simulink model "BarrelControl"  (R2020b)
settings: Solver=VariableStepAuto  StartTime=0.0  StopTime=100  RelTol=1e-3
model workspace (MAT data in the model file):
  C = [0.75  -0.125  -0.5625  0.96875  -0.890625  0.3671875  0.33984375; 1  0  0  0  0  0  0; 0  1  0  0  0  0  0; 0  0  1  0  0  0  0; 0  0  0  1  0  0  0; 0  0  0  0  1  0  0; 0  0  0  0  0  1  0; 0  0  0  0  0  0  1]
  F2Q_xi0 = [1; -1; 1; -1; 1; -1; 1; -1]
  F2Q_xiL = [1; -1; 1; -1; 1; -1; 1; -1]
  Fg = [-29.43; 0; 9.81; 0; 1.962; 0; 0.840857142857; 0]
  Gama = [0  0  0  0  0  0  0; 0  30.2447027552  0  0  0  0  0; 0  0  91.5476694177  0  0  0  0; 0  0  0  175.64612088  0  0  0; 0  0  0  0  277.957713504  0  0; 0  0  0  0  0  1100.88467044  0; 0  0  0  0  0  0  2038.12753726]
  L = 3
  Lambda = [0  0  0  0  0  0  0; 0  91474.204475  0  0  0  0  0; 0  0  838097.577581  0  0  0  0; 0  0  0  3085155.97801  0  0  0; 0  0  0  0  7726049.04966  0  0; 0  0  0  0  0  121194705.761  0; 0  0  0  0  0  0  415396385.815]
  M2Q_xi0 = [0; 0.666666666667; -2.66666666667; 6; -10.6666666667; 16.6666666667; -24; 32.6666666667]
  PHI = [0.136866267704  0.0929914914005  -0.0980787352338  0.0555043868032  -0.144825832461  0.000118902872906  0.118435530445; 0  0.176249339781  -0.0244216885495  -0.133658178847  -0.00189383847447  0.12060390182  0.00720960774598; 0  0.00349791805609  -0.176715791557  -0.00267551593374  -0.105734711917  0.0527964768773  0.110849023327; 0  -0.0152299946368  -0.00490735942162  -0.149265467727  -0.0644504660459  0.117016733417  0.0261303448738; 0  -0.000276595902476  0.0380667589498  0.00904195510557  -0.127293898603  0.0724116243586  0.141528738637; 0  0.00125236425091  0.00154131438463  0.0381220764691  0.018603663864  0.181452010974  0.0171982021012; 0  -6.40906127314e-05  -0.00446596070835  -0.00233149354725  0.0468542529712  0.00391723696732  0.191561402886]
  dpsi_0 = [0; 0.666666666667; -2.66666666667; 6; -10.6666666667; 16.6666666667; -24; 32.6666666667]
  dpsi_L = [0; 0.666666666667; 2.66666666667; 6; 10.6666666667; 16.6666666667; 24; 32.6666666667]
  dpsi_Ldiv8 = [0; 0.666666666667; -2; 2.5; -1; -2.29166666667; 5.625; -6.63541666667]
  psi_0 = [1; -1; 1; -1; 1; -1; 1; -1]
  psi_L = [1; 1; 1; 1; 1; 1; 1; 1]
  ts_controller = 0.001
undefined symbols (not defined in the file): Theta
libraries: cstblocks x4, pid_lib x3, slctrlblks x1, simulink x1
settings Model: EnablePacing=on  OrderedModelArguments=off  Creator=alons  LastModifiedBy=alons

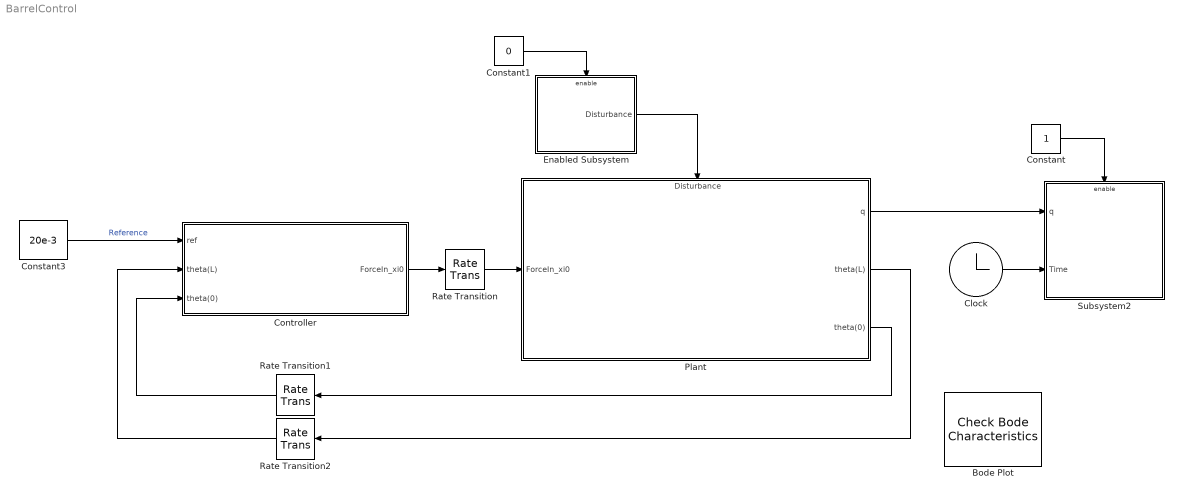
== system BarrelControl ==
  Bode Plot : slctrlblks/Model Verification/Check Bode  Characteristics  InstantiateOnLoad=on  SaveOperatingPoints=off  LinearizationIOs={'/Rate Transition', 1, 'in', 'on', '';'/Plant', 3, 'out', 'on', ''}  LinearizeAt=SnapshotTimes  SnapshotTimes=[0]  TriggerType=rising  SampleTime=auto  RateConversionMethod=zoh  PreWarpFreq=10  UseExactDelayModel=off  UseFullBlockNameLabels=off  UseBusSignalLabels=off  enabled=on  stopWhenAssertionFail=off  export=off  ViewDlgPos=[100 110.6 941 479.4]  OpenViewOnLoad=on  LaunchViewOnOpen=off  FrequencyUnits=rad/s  MagnitudeUnits=dB  PhaseUnits=deg  TimeUnits=seconds  EnableUpperBound=off  UpperBoundFrequencies=[]  UpperBoundMagnitudes=[]  EnableLowerBound=off  LowerBoundFrequencies=[]  LowerBoundMagnitudes=[]
  Clock : Clock
  Constant : Constant  SampleTime=0
      settings: OpenFcn=|
      | if get_param(gcbh,'value')-48
      |    set_param(gcbh,'value','0','backgroundcolor','red');
      | else
      |    set_param(gcbh,'value','1','backgroundcolor','green');
      | end
  Constant1 : Constant  Value=0  SampleTime=0
      settings: OpenFcn=|
      | if get_param(gcbh,'value')-48
      |    set_param(gcbh,'value','0','backgroundcolor','red');
      | else
      |    set_param(gcbh,'value','1','backgroundcolor','green');
      | end
  Constant3 : Constant  Value=20e-3
  Controller : Subsystem  Variant=on  VariantControlMode=label  VariantControl=Choice  LabelModeActiveChoice=Theta(0)
  Enabled Subsystem : Subsystem  TreatAsAtomicUnit=on
  Plant : Subsystem  TreatAsAtomicUnit=on
      settings: PortSchema="{\"entries\":[{\"content\":{\"sides\":[{\"content\":{\"connectorIds\":[\"In1\"]},\"type\":\"ConnectorPlacement.EquallySpacedRectSide\",\"uuid\":\"36edcb47-3a13-438a-ad6c-79b402161546\"},{\"content\":{\"connectorIds\":[\"Out1\",\"Out2\",\"Out3\"],\"side\":\"RIGHT\"},\"type\":\"ConnectorPlacement.EquallySpacedRectSide\",\"uuid\":\"f206446b-0714-4d39-be89-dc03dcd153f7\"},{\"content\":{\"connectorIds\":[\"In2\"],\"side\":\"TOP\"},\"type\":\"ConnectorPlacement.EquallySpacedRectSide\",\"uuid\":\"bd075090-b99d-4803-89e5-3bedf44d599a\"},{\"content\":{\"connectorIds\":[],\"side\":\"HIDDEN\"},\"type\":\"ConnectorPlacement.EquallySpacedRectSide\",\"uuid\":\"510f68a2-1cb4-4401-810b-32bb3d0b381d\"}]},\"type\":\"ConnectorPlacement.EquallySpacedConnector\",\"uuid\":\"6436aeff-31cc-4ec9-a090-95bfbf49f0cf\"}],\"packageUris\":[\"http://schema.mathworks.com/mf0/Connector/R2020b\"],\"version\":\"1.0\"}"
  Rate Transition : RateTransition
  Rate Transition1 : RateTransition  OutPortSampleTime=ts_controller
  Rate Transition2 : RateTransition  OutPortSampleTime=ts_controller
  Subsystem2 : Subsystem
      settings: OpenFcn=|
      | UserData = get_param([gcb,'/AnimationSfcn'],'UserData');
      | Fig = UserData.Figure;
      | if ishghandle(Fig,'figure');
      |    %bring to the front:
      |    figure(Fig);
      | end
      mask Display:
      | t=linspace(0,2*pi,20);
      | plot(cos(t),sin(t));
      | 
      | x=[-0.4,-0.4,0.6,-0.4];
      | y=[-0.5,0.5,0,-0.5];
      | plot(x,y)
      | 
      | color('black');
      | disp('Plot Beam');
  wires:
  Clock/1 -> Subsystem2/2(Time)
  Constant/1 -> Subsystem2/Enable
  Plant/1(q) -> Subsystem2/1(q)
  Plant/2(theta(L)) -> Rate Transition2/1
  Plant/3(theta(0)) -> Rate Transition1/1
  Rate Transition/1 -> Plant/1(ForceIn_xi0)
  Constant3/1 -> Controller/1(ref)  "Reference"
  Rate Transition2/1 -> Controller/2(theta(L))
  Rate Transition1/1 -> Controller/3(theta(0))
  Constant1/1 -> Enabled Subsystem/Enable
  Enabled Subsystem/1(Disturbance) -> Plant/2(Disturbance)
  Controller/1(ForceIn_xi0) -> Rate Transition/1

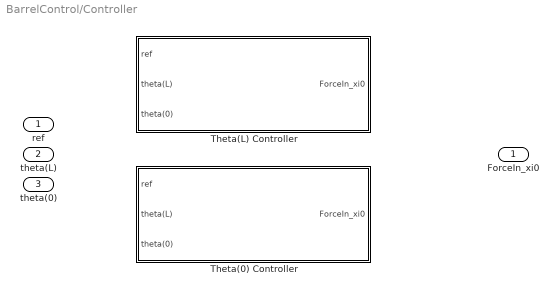
== system BarrelControl/Controller ==
  ref : Inport
  theta(L) : Inport  Port=2
  theta(0) : Inport  Port=3
  Theta(0) Controller : Subsystem  TreatAsAtomicUnit=on  VariantControl=Theta(0)
  Theta(L) Controller : Subsystem  TreatAsAtomicUnit=on  VariantControl=Theta(L)
  ForceIn_xi0 : Outport

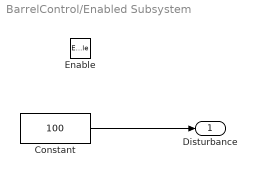
== system BarrelControl/Enabled Subsystem ==
  Enable : EnablePort  StatesWhenEnabling=reset
  Constant : Constant  Value=100
  Disturbance : Outport  OutputWhenDisabled=reset  InitialOutput=0
  wires:
  Constant/1 -> Disturbance/1

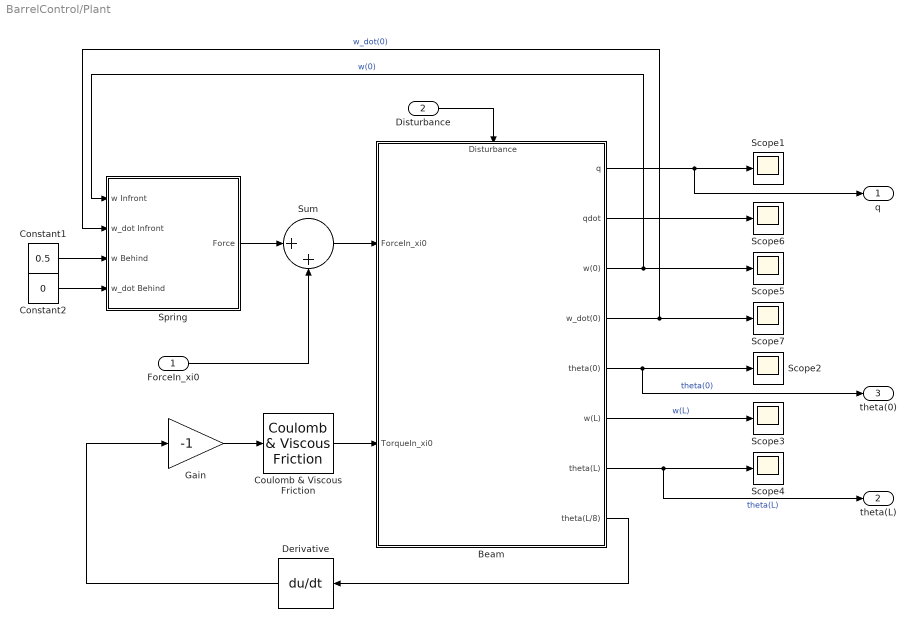
== system BarrelControl/Plant ==
  ForceIn_xi0 : Inport
  Disturbance : Inport  Port=2
  Beam : Subsystem
      settings: PortSchema="{\"entries\":[{\"content\":{\"sides\":[{\"content\":{\"connectorIds\":[\"In1\",\"In2\"]},\"type\":\"ConnectorPlacement.EquallySpacedRectSide\",\"uuid\":\"abe6467a-2196-4326-b3df-78fc9ab57750\"},{\"content\":{\"connectorIds\":[\"Out1\",\"Out2\",\"Out3\",\"Out4\",\"Out5\",\"Out6\",\"Out7\",\"Out8\"],\"side\":\"RIGHT\"},\"type\":\"ConnectorPlacement.EquallySpacedRectSide\",\"uuid\":\"8f33c77a-829a-46db-9e71-a7c761c5b10e\"},{\"content\":{\"connectorIds\":[\"In3\"],\"side\":\"TOP\"},\"type\":\"ConnectorPlacement.EquallySpacedRectSide\",\"uuid\":\"f7becae8-30ec-4352-b968-96f4fe9b45e3\"},{\"content\":{\"connectorIds\":[],\"side\":\"HIDDEN\"},\"type\":\"ConnectorPlacement.EquallySpacedRectSide\",\"uuid\":\"eaf9c01e-636e-4137-bd85-9b7716ad4e28\"}]},\"type\":\"ConnectorPlacement.EquallySpacedConnector\",\"uuid\":\"f90a8ce3-a2cb-42eb-a052-d6f5b77e739e\"}],\"packageUris\":[\"http://schema.mathworks.com/mf0/Connector/R2020b\"],\"version\":\"1.0\"}"
  Constant1 : Constant  Value=0.5
  Constant2 : Constant  Value=0
  Coulomb & Viscous Friction : simulink/Discontinuities/Coulomb & Viscous Friction  offset=15  gain=200
  Derivative : Derivative
  Gain : Gain  Gain=-1
  Scope{1..7} (7 alike) : Scope
  Spring : Subsystem
      mask Display: disp('Spring')
  Sum : Sum  Inputs=|++
  q : Outport
  theta(L) : Outport  Port=2
  theta(0) : Outport  Port=3
  wires:
  Beam/1(q) -> q/1, Scope1/1
  Constant1/1 -> Spring/3(w Behind)
  Beam/2(qdot) -> Scope6/1
  Sum/1 -> Beam/1(ForceIn_xi0)
  Beam/6(w(L)) -> Scope3/1  "w(L)"
  Constant2/1 -> Spring/4(w_dot Behind)
  Spring/1(Force) -> Sum/1
  Beam/3(w(0)) -> Spring/1(w Infront), Scope5/1  "w(0)"
  Beam/7(theta(L)) -> theta(L)/1, Scope4/1  "theta(L)"
  Beam/5(theta(0)) -> theta(0)/1, Scope2/1  "theta(0)"
  Beam/4(w_dot(0)) -> Spring/2(w_dot Infront), Scope7/1  "w_dot(0)"
  Coulomb & Viscous Friction/1 -> Beam/2(TorqueIn_xi0)
  ForceIn_xi0/1 -> Sum/2
  Disturbance/1 -> Beam/3(Disturbance)
  Gain/1 -> Coulomb & Viscous Friction/1
  Beam/8(theta(L/8)) -> Derivative/1
  Derivative/1 -> Gain/1

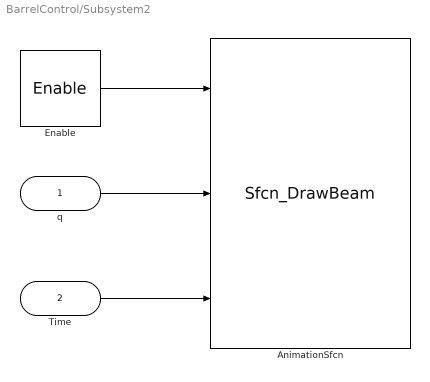
== system BarrelControl/Subsystem2 ==
  q : Inport
  Time : Inport  Port=2
  Enable : EnablePort  StatesWhenEnabling=reset  ShowOutputPort=on
  AnimationSfcn : M-S-Function  FunctionName=Sfcn_DrawBeam  Parameters=L
  wires:
  q/1 -> AnimationSfcn/2
  Enable/1 -> AnimationSfcn/1
  Time/1 -> AnimationSfcn/3

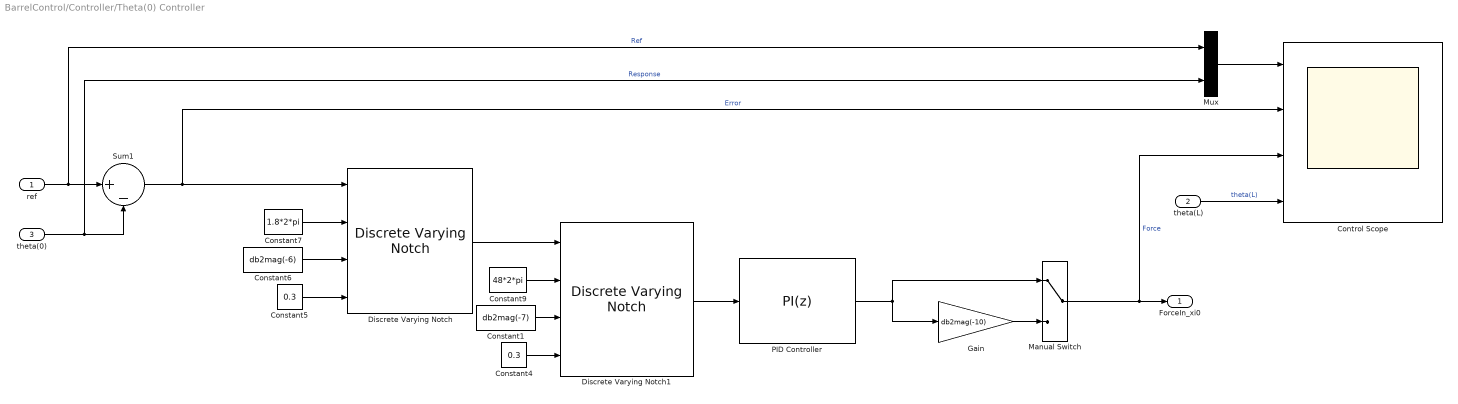
== system BarrelControl/Controller/Theta(0) Controller ==
  ref : Inport
  theta(L) : Inport  Port=2
  theta(0) : Inport  Port=3
  Constant1 : Constant  Value=db2mag(-7)
  Constant4 : Constant  Value=0.3
  Constant5 : Constant  Value=0.3
  Constant6 : Constant  Value=db2mag(-6)
  Constant7 : Constant  Value=1.8*2*pi
  Constant9 : Constant  Value=48*2*pi
  Control Scope : Scope  NumInputPorts=4
  Discrete Varying Notch : cstblocks/Linear Parameter Varying/Discrete Varying Notch  w0=1.5*2*pi  Ts=ts_controller
      settings: SourceProductBaseCode=CT
  Discrete Varying Notch1 : cstblocks/Linear Parameter Varying/Discrete Varying Notch  w0=48*2*pi  Ts=ts_controller
      settings: SourceProductBaseCode=CT
  Gain : Gain  Gain=db2mag(-10)
  Manual Switch : ManualSwitch
  Mux : Mux  Inputs=2
  PID Controller : pid_lib/PID Controller  Controller=PI  Form=Parallel  TimeDomain=Discrete-time  UseExternalTs=off  SampleTime=-1  IntegratorMethod=Forward Euler  FilterMethod=Forward Euler  ControllerParametersSource=internal  P=-9986.27949385  I=-157091.308648994  D=0  UseFilter=on  N=100  TunerSelectOption=Transfer Function Based (PID Tuner App)  InitialConditionSource=internal  InitialConditionForIntegrator=0  InitialConditionForFilter=0  DifferentiatorICPrevScaledInput=0  ExternalReset=none  TrackingMode=off  Kt=1  LimitOutput=off  SatLimitsSource=internal  UpperSaturationLimit=inf  LowerSaturationLimit=-inf  LinearizeAsGain=on  AntiWindupMode=none  Kb=1  POutMin=[]  POutMax=[]  IOutMin=[]  IOutMax=[]  DOutMin=[]  DOutMax=[]  NOutMin=[]  NOutMax=[]  SumOutMin=[]  SumOutMax=[]  SaturationOutMin=[]  SaturationOutMax=[]  PParamMin=[]  PParamMax=[]  IParamMin=[]  IParamMax=[]  DParamMin=[]  DParamMax=[]  NParamMin=[]  NParamMax=[]  KbParamMin=[]  KbParamMax=[]  KtParamMin=[]  KtParamMax=[]  KbOutMin=[]  KbOutMax=[]  KtOutMin=[]  KtOutMax=[]  IntegratorOutMin=[]  IntegratorOutMax=[]  FilterOutMin=[]  FilterOutMax=[]  SumI1OutMin=[]  SumI1OutMax=[]  SumI2OutMin=[]  SumI2OutMax=[]  SumI3OutMin=[]  SumI3OutMax=[]  SumI4OutMin=[]  SumI4OutMax=[]  SumDOutMin=[]  SumDOutMax=[]  DifferentiatorOutMin=[]  DifferentiatorOutMax=[]  FilterDiffOutCoefMin=[]  FilterDiffOutCoefMax=[]  ReciprocalOutMin=[]  ReciprocalOutMax=[]  SumDenOutMin=[]  SumDenOutMax=[]  SumNumOutMin=[]  SumNumOutMax=[]  DivideOutMin=[]  DivideOutMax=[]  UdiffTsProdOutMin=[]  UdiffTsProdOutMax=[]  NTsProdOutMin=[]  NTsProdOutMax=[]  UintegralTsProdOutMin=[]  UintegralTsProdOutMax=[]  UngainTsProdOutMin=[]  UngainTsProdOutMax=[]  IntegratorContinuousStateAttributes=''  IntegratorStateMustResolveToSignalObject=off  IntegratorRTWStateStorageClass=Auto  FilterContinuousStateAttributes=''  FilterStateMustResolveToSignalObject=off  FilterRTWStateStorageClass=Auto  ParallelPVariant=InternalParameters  IdealPVariant=Disabled  IVariant=InternalParameters  DVariant=Disabled  IntegratorVariant=Discrete  SatVariant=Disabled  AWVariant=Passthrough  PCopyVariant=Disabled  TRVariant=Disabled  FdbkBlocksVariant=Forward  IdealPFdbkVariant=Disabled  SatFdbkVariant=Disabled  DerivativeFilterVariant=Disabled  NVariant=Disabled  NCopyVariant=Disabled_SignalSpec  FilterICVariant=Disabled  IntegratorICVariant=InternalICs  ExternalResetVariant=Disabled  TRSumVariant=Passthrough  SumFdbkVariant=Disabled  SumVariant=Sum_PI  TsampFilterVariant=InternalTs  TsampNgainVariant=Passthrough  TsampIntegralVariant=Passthrough  ExternalSaturationOutDataTypeStr=Inherit: Same as second input
  Sum1 : Sum  Inputs=|+-
  ForceIn_xi0 : Outport
  wires:
  theta(0)/1 -> Sum1/2, Mux/2  "Response"
  ref/1 -> Mux/1, Sum1/1  "Ref"
  Constant6/1 -> Discrete Varying Notch/3
  Sum1/1 -> Discrete Varying Notch/1, Control Scope/2  "Error"
  Constant5/1 -> Discrete Varying Notch/4
  Constant7/1 -> Discrete Varying Notch/2
  theta(L)/1 -> Control Scope/4  "theta(L)"
  Constant1/1 -> Discrete Varying Notch1/3
  Constant4/1 -> Discrete Varying Notch1/4
  Constant9/1 -> Discrete Varying Notch1/2
  Mux/1 -> Control Scope/1
  Manual Switch/1 -> Control Scope/3, ForceIn_xi0/1  "Force"
  Gain/1 -> Manual Switch/2
  Discrete Varying Notch/1 -> Discrete Varying Notch1/1
  Discrete Varying Notch1/1 -> PID Controller/1
  PID Controller/1 -> Gain/1, Manual Switch/1

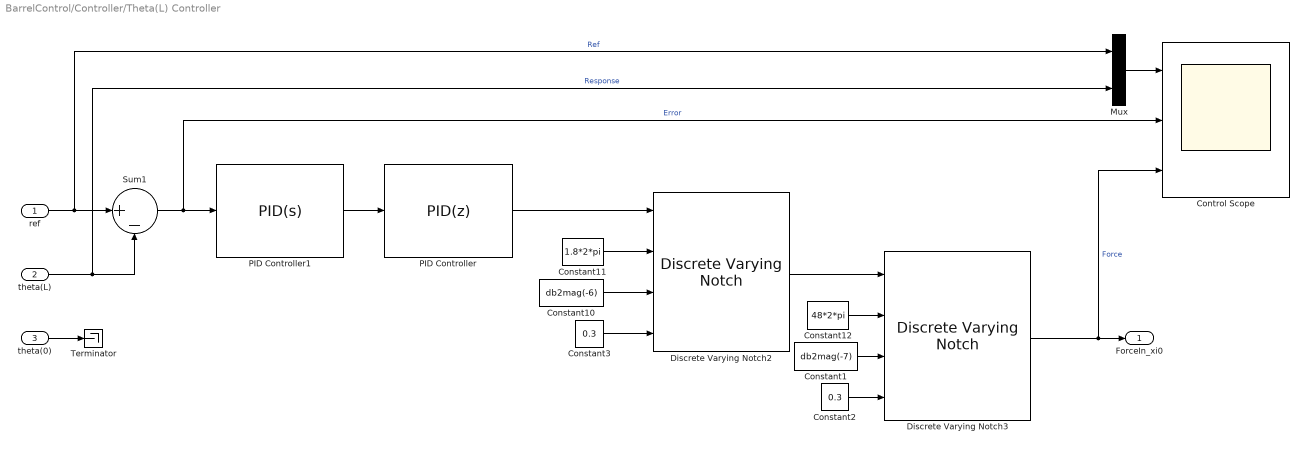
== system BarrelControl/Controller/Theta(L) Controller ==
  ref : Inport
  theta(L) : Inport  Port=2
  theta(0) : Inport  Port=3
  Constant1 : Constant  Value=db2mag(-7)
  Constant10 : Constant  Value=db2mag(-6)
  Constant11 : Constant  Value=1.8*2*pi
  Constant12 : Constant  Value=48*2*pi
  Constant2 : Constant  Value=0.3
  Constant3 : Constant  Value=0.3
  Control Scope : Scope  NumInputPorts=3
  Discrete Varying Notch2 : cstblocks/Linear Parameter Varying/Discrete Varying Notch  w0=1.8*2*pi  Ts=ts_controller
      settings: SourceProductBaseCode=CT
  Discrete Varying Notch3 : cstblocks/Linear Parameter Varying/Discrete Varying Notch  w0=48*2*pi  Ts=ts_controller
      settings: SourceProductBaseCode=CT
  Mux : Mux  Inputs=2
  PID Controller : pid_lib/PID Controller  Controller=PID  Form=Parallel  TimeDomain=Discrete-time  UseExternalTs=off  SampleTime=-1  IntegratorMethod=Forward Euler  FilterMethod=Forward Euler  ControllerParametersSource=internal  P=-0.3*2625.90075309762  I=-0.3*64672.7629914481  D=0  UseFilter=on  N=100  TunerSelectOption=Transfer Function Based (PID Tuner App)  InitialConditionSource=internal  InitialConditionForIntegrator=0  InitialConditionForFilter=0  DifferentiatorICPrevScaledInput=0  ExternalReset=none  TrackingMode=off  Kt=1  LimitOutput=off  SatLimitsSource=internal  UpperSaturationLimit=inf  LowerSaturationLimit=-inf  LinearizeAsGain=on  AntiWindupMode=none  Kb=1  POutMin=[]  POutMax=[]  IOutMin=[]  IOutMax=[]  DOutMin=[]  DOutMax=[]  NOutMin=[]  NOutMax=[]  SumOutMin=[]  SumOutMax=[]  SaturationOutMin=[]  SaturationOutMax=[]  PParamMin=[]  PParamMax=[]  IParamMin=[]  IParamMax=[]  DParamMin=[]  DParamMax=[]  NParamMin=[]  NParamMax=[]  KbParamMin=[]  KbParamMax=[]  KtParamMin=[]  KtParamMax=[]  KbOutMin=[]  KbOutMax=[]  KtOutMin=[]  KtOutMax=[]  IntegratorOutMin=[]  IntegratorOutMax=[]  FilterOutMin=[]  FilterOutMax=[]  SumI1OutMin=[]  SumI1OutMax=[]  SumI2OutMin=[]  SumI2OutMax=[]  SumI3OutMin=[]  SumI3OutMax=[]  SumI4OutMin=[]  SumI4OutMax=[]  SumDOutMin=[]  SumDOutMax=[]  DifferentiatorOutMin=[]  DifferentiatorOutMax=[]  FilterDiffOutCoefMin=[]  FilterDiffOutCoefMax=[]  ReciprocalOutMin=[]  ReciprocalOutMax=[]  SumDenOutMin=[]  SumDenOutMax=[]  SumNumOutMin=[]  SumNumOutMax=[]  DivideOutMin=[]  DivideOutMax=[]  UdiffTsProdOutMin=[]  UdiffTsProdOutMax=[]  NTsProdOutMin=[]  NTsProdOutMax=[]  UintegralTsProdOutMin=[]  UintegralTsProdOutMax=[]  UngainTsProdOutMin=[]  UngainTsProdOutMax=[]  IntegratorContinuousStateAttributes=''  IntegratorStateMustResolveToSignalObject=off  IntegratorRTWStateStorageClass=Auto  FilterContinuousStateAttributes=''  FilterStateMustResolveToSignalObject=off  FilterRTWStateStorageClass=Auto  ParallelPVariant=InternalParameters  IdealPVariant=Disabled  IVariant=InternalParameters  DVariant=InternalParameters  IntegratorVariant=Discrete  SatVariant=Disabled  AWVariant=Passthrough  PCopyVariant=Disabled  TRVariant=Disabled  FdbkBlocksVariant=Forward  IdealPFdbkVariant=Disabled  SatFdbkVariant=Disabled  DerivativeFilterVariant=ForwardEulerFilter  NVariant=InternalParameters  NCopyVariant=Disabled  FilterICVariant=InternalICsFilter  IntegratorICVariant=InternalICs  ExternalResetVariant=Disabled  TRSumVariant=Passthrough  SumFdbkVariant=Disabled  SumVariant=Sum_PID  TsampFilterVariant=InternalTs  TsampNgainVariant=Passthrough  TsampIntegralVariant=Passthrough  ExternalSaturationOutDataTypeStr=Inherit: Same as second input
  PID Controller1 : pid_lib/PID Controller  Controller=PID  Form=Parallel  TimeDomain=Continuous-time  UseExternalTs=off  SampleTime=-1  IntegratorMethod=Forward Euler  FilterMethod=Forward Euler  ControllerParametersSource=internal  P=3.04128238509235  I=0.800754235908562  D=-0.430639702701802  UseFilter=on  N=5.65067418740303  TunerSelectOption=Transfer Function Based (PID Tuner App)  InitialConditionSource=internal  InitialConditionForIntegrator=0  InitialConditionForFilter=0  DifferentiatorICPrevScaledInput=0  ExternalReset=none  TrackingMode=off  Kt=1  LimitOutput=off  SatLimitsSource=internal  UpperSaturationLimit=inf  LowerSaturationLimit=-inf  LinearizeAsGain=on  AntiWindupMode=none  Kb=1  POutMin=[]  POutMax=[]  IOutMin=[]  IOutMax=[]  DOutMin=[]  DOutMax=[]  NOutMin=[]  NOutMax=[]  SumOutMin=[]  SumOutMax=[]  SaturationOutMin=[]  SaturationOutMax=[]  PParamMin=[]  PParamMax=[]  IParamMin=[]  IParamMax=[]  DParamMin=[]  DParamMax=[]  NParamMin=[]  NParamMax=[]  KbParamMin=[]  KbParamMax=[]  KtParamMin=[]  KtParamMax=[]  KbOutMin=[]  KbOutMax=[]  KtOutMin=[]  KtOutMax=[]  IntegratorOutMin=[]  IntegratorOutMax=[]  FilterOutMin=[]  FilterOutMax=[]  SumI1OutMin=[]  SumI1OutMax=[]  SumI2OutMin=[]  SumI2OutMax=[]  SumI3OutMin=[]  SumI3OutMax=[]  SumI4OutMin=[]  SumI4OutMax=[]  SumDOutMin=[]  SumDOutMax=[]  DifferentiatorOutMin=[]  DifferentiatorOutMax=[]  FilterDiffOutCoefMin=[]  FilterDiffOutCoefMax=[]  ReciprocalOutMin=[]  ReciprocalOutMax=[]  SumDenOutMin=[]  SumDenOutMax=[]  SumNumOutMin=[]  SumNumOutMax=[]  DivideOutMin=[]  DivideOutMax=[]  UdiffTsProdOutMin=[]  UdiffTsProdOutMax=[]  NTsProdOutMin=[]  NTsProdOutMax=[]  UintegralTsProdOutMin=[]  UintegralTsProdOutMax=[]  UngainTsProdOutMin=[]  UngainTsProdOutMax=[]  IntegratorContinuousStateAttributes=''  IntegratorStateMustResolveToSignalObject=off  IntegratorRTWStateStorageClass=Auto  FilterContinuousStateAttributes=''  FilterStateMustResolveToSignalObject=off  FilterRTWStateStorageClass=Auto  ParallelPVariant=InternalParameters  IdealPVariant=Disabled  IVariant=InternalParameters  DVariant=InternalParameters  IntegratorVariant=Continuous  SatVariant=Disabled  AWVariant=Passthrough  PCopyVariant=Disabled  TRVariant=Disabled  FdbkBlocksVariant=Forward  IdealPFdbkVariant=Disabled  SatFdbkVariant=Disabled  DerivativeFilterVariant=ContFilter  NVariant=InternalParameters  NCopyVariant=Disabled  FilterICVariant=InternalICsFilter  IntegratorICVariant=InternalICs  ExternalResetVariant=Disabled  TRSumVariant=Passthrough  SumFdbkVariant=Disabled  SumVariant=Sum_PID  TsampFilterVariant=InternalTs  TsampNgainVariant=Passthrough  TsampIntegralVariant=Passthrough  ExternalSaturationOutDataTypeStr=Inherit: Same as second input
  Sum1 : Sum  Inputs=|+-
  Terminator : Terminator
  ForceIn_xi0 : Outport
  wires:
  Discrete Varying Notch3/1 -> Control Scope/3, ForceIn_xi0/1  "Force"
  PID Controller1/1 -> PID Controller/1
  Sum1/1 -> Control Scope/2, PID Controller1/1  "Error"
  ref/1 -> Mux/1, Sum1/1  "Ref"
  theta(L)/1 -> Mux/2, Sum1/2  "Response"
  theta(0)/1 -> Terminator/1
  Mux/1 -> Control Scope/1
  PID Controller/1 -> Discrete Varying Notch2/1
  Constant12/1 -> Discrete Varying Notch3/2
  Constant2/1 -> Discrete Varying Notch3/4
  Constant11/1 -> Discrete Varying Notch2/2
  Constant3/1 -> Discrete Varying Notch2/4
  Constant1/1 -> Discrete Varying Notch3/3
  Constant10/1 -> Discrete Varying Notch2/3
  Discrete Varying Notch2/1 -> Discrete Varying Notch3/1

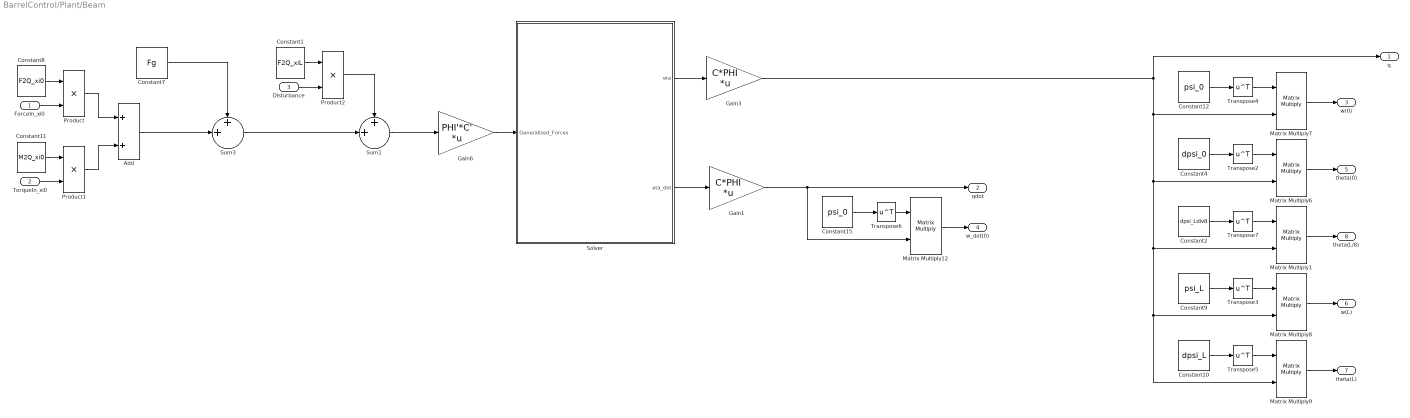
== system BarrelControl/Plant/Beam ==
  ForceIn_xi0 : Inport
  TorqueIn_xi0 : Inport  Port=2
  Disturbance : Inport  Port=3
  Add : Sum
  Constant1 : Constant  Value=F2Q_xiL
  Constant10 : Constant  Value=dpsi_L
  Constant11 : Constant  Value=M2Q_xi0
  Constant12 : Constant  Value=psi_0
  Constant15 : Constant  Value=psi_0
  Constant2 : Constant  Value=dpsi_Ldiv8
  Constant4 : Constant  Value=dpsi_0
  Constant7 : Constant  Value=Fg
  Constant8 : Constant  Value=F2Q_xi0
  Constant9 : Constant  Value=psi_L
  Gain1 : Gain  Gain=C*PHI  Multiplication=Matrix(K*u) (u vector)
  Gain3 : Gain  Gain=C*PHI  Multiplication=Matrix(K*u) (u vector)
  Gain6 : Gain  Gain=PHI'*C'  Multiplication=Matrix(K*u) (u vector)
  Matrix Multiply{1,6..9,12} (6 alike) : Product  Multiplication=Matrix(*)
  Product : Product
  Product1 : Product
  Product2 : Product
  Solver : Subsystem  TreatAsAtomicUnit=on
  Sum1 : Sum  Inputs=++|
  Sum3 : Sum  Inputs=++|
  Transpose{2..7} (6 alike) : Math  Operator=transpose  SaturateOnIntegerOverflow=on
  q : Outport
  qdot : Outport  Port=2
  w(0) : Outport  Port=3
  w_dot(0) : Outport  Port=4
  theta(0) : Outport  Port=5
  w(L) : Outport  Port=6
  theta(L) : Outport  Port=7
  theta(L/8) : Outport  Port=8
  wires:
  Constant4/1 -> Transpose2/1
  Transpose2/1 -> Matrix Multiply6/1
  Matrix Multiply6/1 -> theta(0)/1
  Add/1 -> Sum3/2
  Constant10/1 -> Transpose5/1
  Transpose3/1 -> Matrix Multiply8/1
  Transpose5/1 -> Matrix Multiply9/1
  Constant9/1 -> Transpose3/1
  Matrix Multiply9/1 -> theta(L)/1
  Matrix Multiply8/1 -> w(L)/1
  Constant7/1 -> Sum3/1
  Constant8/1 -> Product/1
  ForceIn_xi0/1 -> Product/2
  TorqueIn_xi0/1 -> Product1/2
  Constant11/1 -> Product1/1
  Product1/1 -> Add/2
  Product/1 -> Add/1
  Transpose4/1 -> Matrix Multiply7/1
  Constant12/1 -> Transpose4/1
  Matrix Multiply7/1 -> w(0)/1
  Constant15/1 -> Transpose6/1
  Transpose6/1 -> Matrix Multiply12/1
  Matrix Multiply12/1 -> w_dot(0)/1
  Solver/2(eta_dot) -> Gain1/1
  Constant1/1 -> Product2/1
  Disturbance/1 -> Product2/2
  Sum3/1 -> Sum1/2
  Product2/1 -> Sum1/1
  Constant2/1 -> Transpose7/1
  Matrix Multiply1/1 -> theta(L/8)/1
  Transpose7/1 -> Matrix Multiply1/1
  Solver/1(eta) -> Gain3/1
  Gain3/1 -> q/1, Matrix Multiply7/2, Matrix Multiply1/2, Matrix Multiply9/2, Matrix Multiply8/2, Matrix Multiply6/2
  Gain1/1 -> qdot/1, Matrix Multiply12/2
  Sum1/1 -> Gain6/1
  Gain6/1 -> Solver/1(Generalized_Forces)

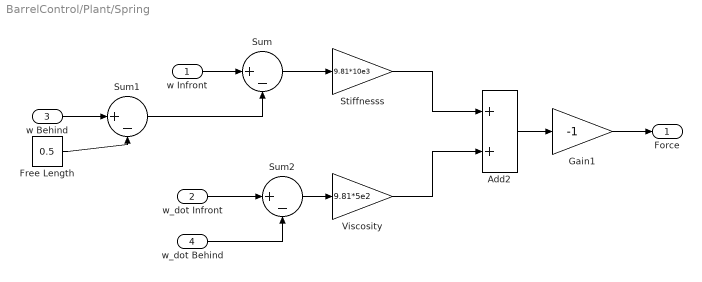
== system BarrelControl/Plant/Spring ==
  w Infront : Inport
  w_dot Infront : Inport  Port=2
  w Behind : Inport  Port=3
  w_dot Behind : Inport  Port=4
  Add2 : Sum
  Free Length : Constant  Value=0.5
  Gain1 : Gain  Gain=-1
  Stiffnesss : Gain  Gain=9.81*10e3
  Sum : Sum  Inputs=|+-
  Sum1 : Sum  Inputs=|+-
  Sum2 : Sum  Inputs=|+-
  Viscosity : Gain  Gain=9.81*5e2
  Force : Outport
  wires:
  w Infront/1 -> Sum/1
  Sum/1 -> Stiffnesss/1
  w_dot Behind/1 -> Sum2/2
  w_dot Infront/1 -> Sum2/1
  Add2/1 -> Gain1/1
  Stiffnesss/1 -> Add2/1
  Sum2/1 -> Viscosity/1
  Gain1/1 -> Force/1
  Viscosity/1 -> Add2/2
  w Behind/1 -> Sum1/1
  Free Length/1 -> Sum1/2
  Sum1/1 -> Sum/2

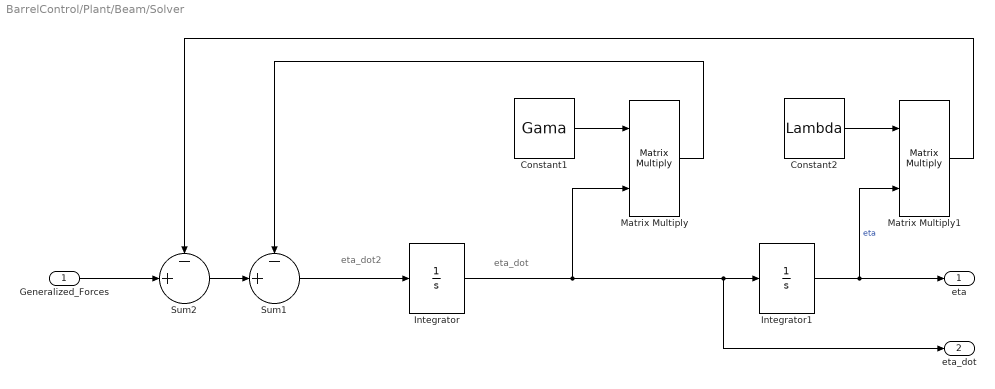
== system BarrelControl/Plant/Beam/Solver ==
  note: eta_dot2
  note: eta_dot
  Generalized_Forces : Inport
  Constant1 : Constant  Value=Gama
  Constant2 : Constant  Value=Lambda
  Integrator : Integrator
  Integrator1 : Integrator
  Matrix Multiply : Product  Multiplication=Matrix(*)
  Matrix Multiply1 : Product  Multiplication=Matrix(*)
  Sum1 : Sum  Inputs=-+|
  Sum2 : Sum  Inputs=-+|
  eta : Outport
  eta_dot : Outport  Port=2
  wires:
  Constant1/1 -> Matrix Multiply/1
  Integrator/1 -> Integrator1/1, eta_dot/1, Matrix Multiply/2
  Sum1/1 -> Integrator/1
  Constant2/1 -> Matrix Multiply1/1
  Matrix Multiply1/1 -> Sum2/1
  Integrator1/1 -> eta/1, Matrix Multiply1/2  "eta"
  Matrix Multiply/1 -> Sum1/1
  Sum2/1 -> Sum1/2
  Generalized_Forces/1 -> Sum2/2
